simulink model "modelo_rk4"  (R2025a)
settings: Solver=FixedStepDiscrete  StartTime=0.0  StopTime=tf  FixedStep=h  RelTol=1e-3
values from neighbouring files (symbols this model uses):
  h = 0.1    [ejemplo_NOlineal_RK4.m]    (also in euler_explicita.m = (tf - t0)/n; euler_explicito.m = (tf - t0)/n; euler_midpoint.m = (tf - t0)/n; examplecrk4.m)
  y0 = 1    [ExampleEuler.m]    (also in ejemplo_NOlineal_RK4.m; examplecrk4.m; exmapleEuler2.m; lineal_RK4.m)
undefined symbols (not defined in the file or in its folder): rk4_step
settings Model: Creator=a.diteodoro  LastModifiedBy=a.diteodoro

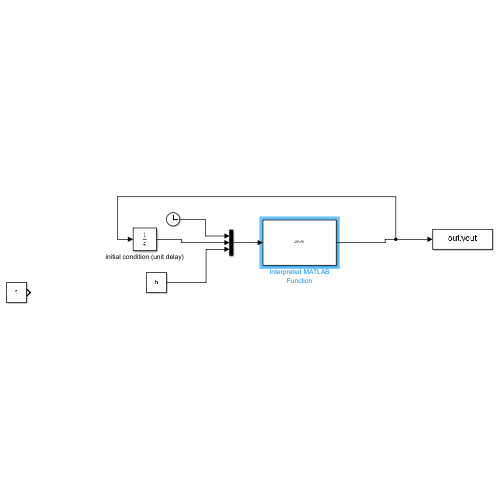
[thumbnail: Simulink's stored preview of the top-level diagram]
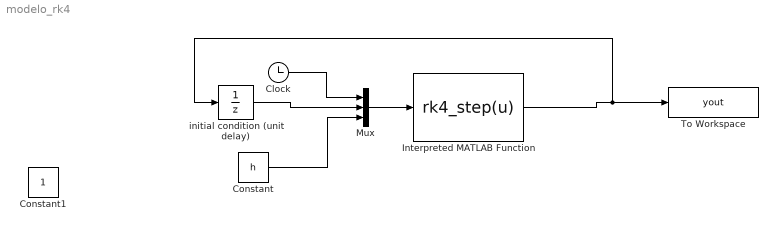
== system modelo_rk4 ==
  Clock : Clock
  Constant : Constant  Value=h
  Constant1 : Constant
  Interpreted MATLAB Function : MATLABFcn  MATLABFcn=rk4_step(u)
  Mux : Mux  Inputs=3
  To Workspace : ToWorkspace  VariableName=yout  SaveFormat=Structure With Time  SampleTime=-1
  initial condition (unit delay) : UnitDelay  InitialCondition=y0  SampleTime=-1  HasFrameUpgradeWarning=on
  wires:
  Clock/1 -> Mux/1
  Interpreted MATLAB Function/1 -> initial condition (unit delay)/1, To Workspace/1
  Mux/1 -> Interpreted MATLAB Function/1
  initial condition (unit delay)/1 -> Mux/2
  Constant/1 -> Mux/3
